simulink subsystem "ttc_on_road"  (R2022b)
settings: Solver=VariableStepAuto  StartTime=0.0  StopTime=10.0  RelTol=1e-3
settings Model: Creator=USER  LastModifiedBy=User

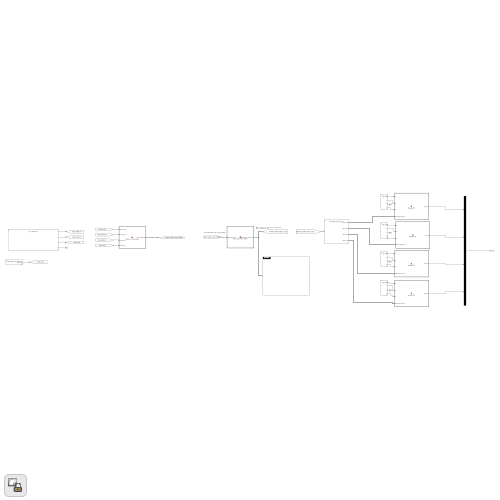
[thumbnail: Simulink's stored preview of the top-level diagram]
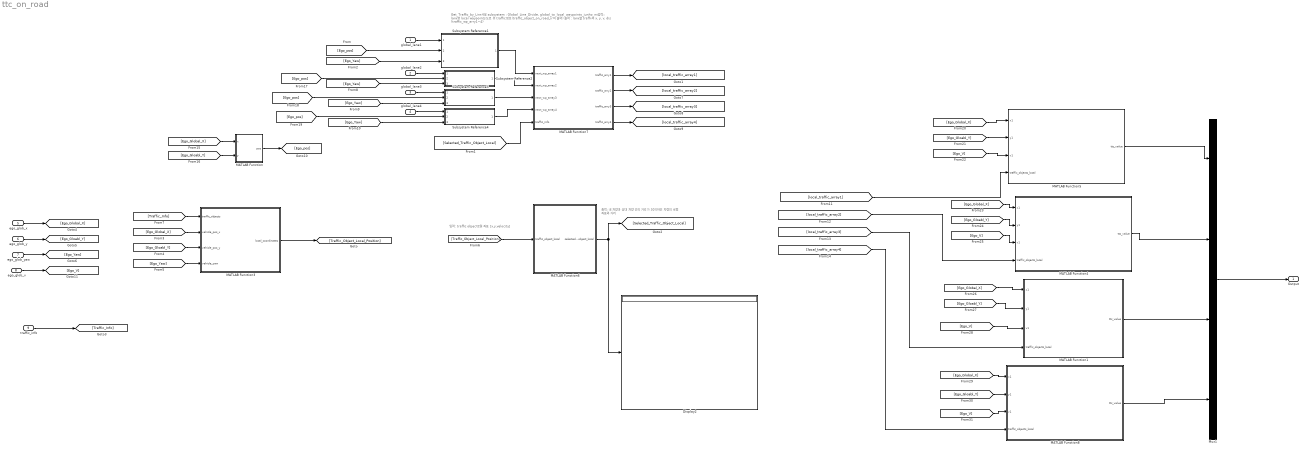
== system ttc_on_road ==
  note: 입력: traffic object 로컬 좌표 [x,y,velocity]
  note: 출력: 내 차량과 상대 차량 간의 거리가 30이하인 차령의 로컬 좌표와 거리
  note: Get_Traffic_by_Line(사용 subsystem : Global_Line_Divide, global_to_local_waypoints_junho_new) :
      | 입력 : lane별 local waypoints, 도로 위 traffic 정보(traffic_object_on_road_info의 출력)
      | 출력 : lane별 traffic의 x, y, v, dis (traffic_wp_arry1~4)
  global_lane1 : Inport
  global_lane2 : Inport  Port=2
  global_lane3 : Inport  Port=3
  global_lane4 : Inport  Port=4
  ego_glob_x : Inport  Port=5
  ego_glob_y : Inport  Port=6
  ego_glob_yaw : Inport  Port=7
  ego_glob_v : Inport  Port=8
  traffic_info : Inport  Port=9
  Display2 : Display
  MATLAB Function : MATLAB Function  TreatAsAtomicUnit=on
  MATLAB Function1 : MATLAB Function  TreatAsAtomicUnit=on
  MATLAB Function3 : MATLAB Function  TreatAsAtomicUnit=on
  MATLAB Function4 : MATLAB Function  TreatAsAtomicUnit=on
  MATLAB Function5 : MATLAB Function  TreatAsAtomicUnit=on
  MATLAB Function6 : MATLAB Function  TreatAsAtomicUnit=on
  MATLAB Function7 : MATLAB Function  TreatAsAtomicUnit=on
  MATLAB Function8 : MATLAB Function  TreatAsAtomicUnit=on
  Mux1 : Mux
  Subsystem Reference{1..4} (4 alike) : Subsystem  ReferencedSubsystem=global_to_local_waypoint_junho
  Output : Outport
  wires:
  traffic_info/1 -> [Traffic_Info]
  ego_glob_yaw/1 -> [Ego_Yaw]
  MATLAB Function6/1(selected_traffic_object_local) -> [Selected_Traffic_Object_Local], Display2/1
  [Ego_Gloabl_Y] -> MATLAB Function3/3(vehicle_pos_y)
  ego_glob_x/1 -> [Ego_Global_X]
  MATLAB Function1/1(ttc_value) -> Mux1/3
  [Ego_Yaw] -> MATLAB Function3/4(vehicle_yaw)
  [Traffic_Info] -> MATLAB Function3/1(traffic_objects)
  ego_glob_y/1 -> [Ego_Gloabl_Y]
  Mux1/1 -> Output/1
  MATLAB Function3/1(local_coordinates) -> [Traffic_Object_Local_Position]
  [Traffic_Object_Local_Position] -> MATLAB Function6/1(traffic_object_local)
  [local_traffic_array2] -> MATLAB Function4/4(traffic_objects_local)
  [Ego_Global_X] -> MATLAB Function3/2(vehicle_pos_x)
  MATLAB Function5/1(ttc_value) -> Mux1/1
  [local_traffic_array3] -> MATLAB Function1/4(traffic_objects_local)
  MATLAB Function8/1(ttc_value) -> Mux1/4
  [local_traffic_array1] -> MATLAB Function5/4(traffic_objects_local)
  [local_traffic_array4] -> MATLAB Function8/4(traffic_objects_local)
  MATLAB Function4/1(ttc_value) -> Mux1/2
  MATLAB Function7/3(traffic_arry3) -> [local_traffic_array3]
  Subsystem Reference3/1 -> MATLAB Function7/3(next_wp_array3)
  Subsystem Reference2/1 -> MATLAB Function7/2(next_wp_array2)
  MATLAB Function7/2(traffic_arry2) -> [local_traffic_array2]
  Subsystem Reference1/1 -> MATLAB Function7/1(next_wp_array1)
  Subsystem Reference4/1 -> MATLAB Function7/4(next_wp_array4)
  MATLAB Function7/4(traffic_arry4) -> [local_traffic_array4]
  MATLAB Function7/1(traffic_arry1) -> [local_traffic_array1]
  [Selected_Traffic_Object_Local] -> MATLAB Function7/5(traffic_info)
  global_lane1/1 -> Subsystem Reference1/1
  global_lane2/1 -> Subsystem Reference2/1
  global_lane3/1 -> Subsystem Reference3/1
  global_lane4/1 -> Subsystem Reference4/1
  [Ego_Yaw] -> Subsystem Reference1/3
  [Ego_Yaw] -> Subsystem Reference2/3
  [Ego_Yaw] -> Subsystem Reference3/3
  [Ego_Yaw] -> Subsystem Reference4/3
  [Ego_Global_X] -> MATLAB Function/1(x)
  [Ego_Gloabl_Y] -> MATLAB Function/2(y)
  MATLAB Function/1(pos) -> [Ego_pos]
  [Ego_pos] -> Subsystem Reference1/2
  [Ego_pos] -> Subsystem Reference2/2
  [Ego_pos] -> Subsystem Reference3/2
  [Ego_pos] -> Subsystem Reference4/2
  [Ego_Global_X] -> MATLAB Function5/1(x1)
  [Ego_Gloabl_Y] -> MATLAB Function5/2(y1)
  [Ego_V] -> MATLAB Function5/3(v1)
  ego_glob_v/1 -> [Ego_V]
  [Ego_Global_X] -> MATLAB Function4/1(x1)
  [Ego_Gloabl_Y] -> MATLAB Function4/2(y1)
  [Ego_V] -> MATLAB Function4/3(v1)
  [Ego_Global_X] -> MATLAB Function1/1(x1)
  [Ego_Gloabl_Y] -> MATLAB Function1/2(y1)
  [Ego_Global_X] -> MATLAB Function8/1(x1)
  [Ego_Gloabl_Y] -> MATLAB Function8/2(y1)
  [Ego_V] -> MATLAB Function8/3(v1)
  [Ego_V] -> MATLAB Function1/3(v1)

== matlab function ttc_on_road/MATLAB Function3 ==
  data: traffic_objects input; local_coordinates output; vehicle_pos_x input; vehicle_pos_y input; vehicle_yaw input
function local_coordinates = global_to_local_position(traffic_objects, vehicle_pos_x, vehicle_pos_y, vehicle_yaw)
    % 가변 크기를 [30, 3]로 설정 (최대 30개의 객체를 지원)
    local_coordinates = zeros(30, 3);  % 초기화 시 고정 크기로 배열 생성

    % 차량 위치를 기준으로 변환 (평행 이동)
    delta_x = traffic_objects(:, 1) - vehicle_pos_x;
    delta_y = traffic_objects(:, 2) - vehicle_pos_y;

    % 차량의 요(방향)에 따른 회전 변환
    x_l = cos(vehicle_yaw) * delta_x + sin(vehicle_yaw) * delta_y;
    y_l = -sin(vehicle_yaw) * delta_x + cos(vehicle_yaw) * delta_y;

    % 유효한 객체의 수만큼 지역 좌표를 저장
    num_objects = min(size(traffic_objects, 1), 30); % 최대 30개의 객체로 제한

    for i = 1:num_objects
        velocity = sqrt(traffic_objects(i, 3)^2 + traffic_objects(i, 4)^2);
        local_coordinates(i, :) = [x_l(i), y_l(i), velocity];
    end

    % 나머지 행은 NaN으로 채워 고정 크기 배열 유지
    if num_objects < 30
        local_coordinates(num_objects+1:end, :) = NaN;
    end
end

== matlab function ttc_on_road/MATLAB Function1 ==
  data: x1 input; ttc_value output; y1 input; v1 input; traffic_objects_local input
function ttc_value = calculateTTC(x1, y1, v1, traffic_objects_local)
    % 여러 상대 차량과의 Time to Collision 계산 함수
    % 입력:
    %   x1, y1 - 내 차량의 좌표
    %   v1 - 내 차량의 속도 (크기)
    %   traffic_objects_local - Nx3 행렬로, 각 행은 상대 차량의 (x, y,velocity) 좌표
    %   distance - Nx1 벡터로 내 차량과 다른 차량 사이의 거리
    % 출력:
    %   ttc_values - 각 상대 차량과의 Time to Collision 값

    % 차량 수
    numVehicles = size(traffic_objects_local, 1);

    if numVehicles > 0
        % 거리 및 TTC 저장을 위한 배열 초기화
        ttc_values = zeros(numVehicles, 1);
        
        % 각 차량과의 거리 및 상대 속도 계산
        for i = 1:numVehicles
    
            % 상대 속도 계산 (내 차량 속도와 상대 차량 속도의 차이)
            v2 = traffic_objects_local(i,3);
            relative_velocity = v2 - v1;
            temp_ttc = traffic_objects_local(i,4) / relative_velocity; 
            % Time to Collision 계산
            ttc_values(i) = abs(traffic_objects_local(i,4) / relative_velocity);
        end

        % 행렬에서 inf 값을 제외한 값들만 선택
        finiteValues = ttc_values(isfinite(ttc_values));
    
        % inf가 아닌 값들 중 최소 값 계산
        if ~isempty(finiteValues)
            ttc_value = min(finiteValues);
        else
            % 모든 값이 inf일 경우
            ttc_value = inf;
        end
    
    else
        ttc_value = inf;
    end
end

== matlab function ttc_on_road/MATLAB Function4 ==
  data: x1 input; ttc_value output; y1 input; v1 input; traffic_objects_local input
function ttc_value = calculateTTC(x1, y1, v1, traffic_objects_local)
    % 여러 상대 차량과의 Time to Collision 계산 함수
    % 입력:
    %   x1, y1 - 내 차량의 좌표
    %   v1 - 내 차량의 속도 (크기)
    %   traffic_objects_local - Nx3 행렬로, 각 행은 상대 차량의 (x, y,velocity) 좌표
    %   distance - Nx1 벡터로 내 차량과 다른 차량 사이의 거리
    % 출력:
    %   ttc_values - 각 상대 차량과의 Time to Collision 값

    % 차량 수
    numVehicles = size(traffic_objects_local, 1);

    if numVehicles > 0
        % 거리 및 TTC 저장을 위한 배열 초기화
        ttc_values = zeros(numVehicles, 1);
        
        % 각 차량과의 거리 및 상대 속도 계산
        for i = 1:numVehicles
    
            % 상대 속도 계산 (내 차량 속도와 상대 차량 속도의 차이)
            v2 = traffic_objects_local(i,3);
            relative_velocity = v2 - v1;
            temp_ttc = traffic_objects_local(i,4) / relative_velocity; 
            % Time to Collision 계산
            ttc_values(i) = abs(traffic_objects_local(i,4) / relative_velocity);
        end

        % 행렬에서 inf 값을 제외한 값들만 선택
        finiteValues = ttc_values(isfinite(ttc_values));
    
        % inf가 아닌 값들 중 최소 값 계산
        if ~isempty(finiteValues)
            ttc_value = min(finiteValues);
        else
            % 모든 값이 inf일 경우
            ttc_value = inf;
        end
    
    else
        ttc_value = inf;
    end
end

== matlab function ttc_on_road/MATLAB Function5 ==
  data: x1 input; ttc_value output; y1 input; v1 input; traffic_objects_local input
function ttc_value = calculateTTC(x1, y1, v1, traffic_objects_local)
    % 여러 상대 차량과의 Time to Collision 계산 함수
    % 입력:
    %   x1, y1 - 내 차량의 좌표
    %   v1 - 내 차량의 속도 (크기)
    %   traffic_objects_local - Nx3 행렬로, 각 행은 상대 차량의 (x, y,velocity) 좌표
    %   distance - Nx1 벡터로 내 차량과 다른 차량 사이의 거리
    % 출력:
    %   ttc_values - 각 상대 차량과의 Time to Collision 값

    % 차량 수
    numVehicles = size(traffic_objects_local, 1);

    if numVehicles > 0
        % 거리 및 TTC 저장을 위한 배열 초기화
        ttc_values = zeros(numVehicles, 1);
        
        % 각 차량과의 거리 및 상대 속도 계산
        for i = 1:numVehicles
    
            % 상대 속도 계산 (내 차량 속도와 상대 차량 속도의 차이)
            v2 = traffic_objects_local(i,3);
            relative_velocity = v2 - v1;
            temp_ttc = traffic_objects_local(i,4) / relative_velocity; 
            % Time to Collision 계산
            ttc_values(i) = abs(traffic_objects_local(i,4) / relative_velocity);
        end

        % 행렬에서 inf 값을 제외한 값들만 선택
        finiteValues = ttc_values(isfinite(ttc_values));
    
        % inf가 아닌 값들 중 최소 값 계산
        if ~isempty(finiteValues)
            ttc_value = min(finiteValues);
        else
            % 모든 값이 inf일 경우
            ttc_value = inf;
        end
    
    else
        ttc_value = inf;
    end
end

== matlab function ttc_on_road/MATLAB Function6 ==
  data: traffic_object_local input; selected_traffic_object_local output
function selected_traffic_object_local = select_near_traffic_object(traffic_object_local)
    % 차량 수
    numVehicles = size(traffic_object_local, 1);
    
    % 가변 크기 설정: 최대 30x4 크기
    selected_traffic_object_local = zeros(30, 4); 

    count = 1; % 유효 객체 카운터

    % 각 차량과의 거리 계산 및 거리가 30이하인 경우 선택
    for i = 1:numVehicles
        x = traffic_object_local(i,1);
        y = traffic_object_local(i,2);
        distance = sqrt(x^2 + y^2) - 4.47;

        if distance <= 30
            % 거리 조건에 맞는 traffic object만 배열에 추가
            selected_traffic_object_local(count, :) = [traffic_object_local(i, :), distance];
            count = count + 1;
            
            % 최대 크기를 넘지 않도록 설정
            if count > 30
                break;
            end
        end
    end
    
    % 남은 행들을 NaN으로 채워 고정 크기로 유지
    if count <= 30
        selected_traffic_object_local(count:end, :) = NaN;
    end
end

== matlab function ttc_on_road/MATLAB Function ==
  data: x input; pos output; y input
function pos = xy_2_pos(x, y)

    pos = [x,y];

end

== matlab function ttc_on_road/MATLAB Function8 ==
  data: x1 input; ttc_value output; y1 input; v1 input; traffic_objects_local input
function ttc_value = calculateTTC(x1, y1, v1, traffic_objects_local)
    % 여러 상대 차량과의 Time to Collision 계산 함수
    % 입력:
    %   x1, y1 - 내 차량의 좌표
    %   v1 - 내 차량의 속도 (크기)
    %   traffic_objects_local - Nx3 행렬로, 각 행은 상대 차량의 (x, y,velocity) 좌표
    %   distance - Nx1 벡터로 내 차량과 다른 차량 사이의 거리
    % 출력:
    %   ttc_values - 각 상대 차량과의 Time to Collision 값

    % 차량 수
    numVehicles = size(traffic_objects_local, 1);

    if numVehicles > 0
        % 거리 및 TTC 저장을 위한 배열 초기화
        ttc_values = zeros(numVehicles, 1);
        
        % 각 차량과의 거리 및 상대 속도 계산
        for i = 1:numVehicles
    
            % 상대 속도 계산 (내 차량 속도와 상대 차량 속도의 차이)
            v2 = traffic_objects_local(i,3);
            relative_velocity = v2 - v1;
            temp_ttc = traffic_objects_local(i,4) / relative_velocity; 
            % Time to Collision 계산
            ttc_values(i) = abs(traffic_objects_local(i,4) / relative_velocity);
        end

        % 행렬에서 inf 값을 제외한 값들만 선택
        finiteValues = ttc_values(isfinite(ttc_values));
    
        % inf가 아닌 값들 중 최소 값 계산
        if ~isempty(finiteValues)
            ttc_value = min(finiteValues);
        else
            % 모든 값이 inf일 경우
            ttc_value = inf;
        end
    
    else
        ttc_value = inf;
    end
end

== matlab function ttc_on_road/MATLAB Function7 ==
  settings: sampleTime=0.001
  data: next_wp_array1 input; next_wp_array2 input; next_wp_array3 input; next_wp_array4 input; traffic_arry1 output size=[8 4]; traffic_info input; traffic_arry2 output size=[8 4]; traffic_arry3 output size=[8 4]; traffic_arry4 output size=[8 4]
function [traffic_arry1, traffic_arry2, traffic_arry3, traffic_arry4] = get_traffic(next_wp_array1, next_wp_array2, next_wp_array3, next_wp_array4, traffic_info)
    tolerance = 3; % 트래픽 위치에 대한 오차 허용 범위

    % Initialize traffic waypoints array with NaNs (size 8x4 to limit maximum size)
    coder.varsize('traffic_arry1', [8, 4]);  % 행은 8로 설정, 열은 4로 고정
    traffic_arry1 = zeros(0,4);
    coder.varsize('traffic_arry2', [8, 4]);  % 행은 8로 설정, 열은 4로 고정
    traffic_arry2 = zeros(0,4);
    coder.varsize('traffic_arry3', [8, 4]);  % 행은 8로 설정, 열은 4로 고정
    traffic_arry3 = zeros(0,4);
    coder.varsize('traffic_arry4', [8, 4]);  % 행은 8로 설정, 열은 4로 고정
    traffic_arry4 = zeros(0,4);

    % 트래픽 정보를 각 lane의 waypoints와 비교하여 저장
    for i = 1:size(traffic_info, 1) % 각 트래픽 정보에 대해 반복
        traffic_x = traffic_info(i, 1);
        traffic_y = traffic_info(i, 2);
        traffic_v = traffic_info(i, 3);
        traffic_dis = traffic_info(i, 4);

        % 각 lane의 waypoints와 트래픽 위치 비교 (오차 tolerance 범위 내)
        if is_within_tolerance(traffic_x, traffic_y, next_wp_array1, tolerance)
            traffic_arry1 = add_to_traffic_array(traffic_arry1, [traffic_x, traffic_y, traffic_v, traffic_dis]);
        elseif is_within_tolerance(traffic_x, traffic_y, next_wp_array2, tolerance)
            traffic_arry2 = add_to_traffic_array(traffic_arry2, [traffic_x, traffic_y, traffic_v, traffic_dis]);
        elseif is_within_tolerance(traffic_x, traffic_y, next_wp_array3, tolerance)
            traffic_arry3 = add_to_traffic_array(traffic_arry3, [traffic_x, traffic_y, traffic_v, traffic_dis]);
        elseif is_within_tolerance(traffic_x, traffic_y, next_wp_array4, tolerance)
            traffic_arry4 = add_to_traffic_array(traffic_arry4, [traffic_x, traffic_y, traffic_v, traffic_dis]);
        end
    end
end

% 트래픽 좌표가 해당 lane의 waypoints와 오차 tolerance 범위 내에 있는지 확인하는 함수
function is_within = is_within_tolerance(traffic_x, traffic_y, waypoints, tolerance)
    distances = sqrt((waypoints(:, 1) - traffic_x).^2 + (waypoints(:, 2) - traffic_y).^2);
    is_within = any(distances <= tolerance); % 오차 tolerance 이내에 있는지 확인
end

% 트래픽 정보를 해당 lane array에 추가하는 함수
function updated_array = add_to_traffic_array(traffic_array, traffic_data)
    % 배열의 크기를 제한 (최대 8x4)
    if size(traffic_array, 1) < 8
        % 현재 배열에 행 추가
        traffic_array = [traffic_array; traffic_data];
    end
    updated_array = traffic_array;
end
